simulink model "Controlled_Motor_Position"  (R2020b)
settings: Solver=VariableStepAuto  StartTime=0.0  StopTime=10.0  RelTol=1e-3
values from neighbouring files (symbols this model uses):
  b = 3.5077E-6    [data.sldd]
  J = 3.2284E-6    [data.sldd]
  K = 0.0274    [data.sldd]
  Kd = 0.04    [data.sldd]
  Ki = 47.4    [data.sldd]
  Kp = 3.4    [data.sldd]
  L = 2.75E-6    [data.sldd]
  R = 4.0    [data.sldd]
settings Model: DataDictionary=data.sldd  Creator=vikas  LastModifiedBy=family

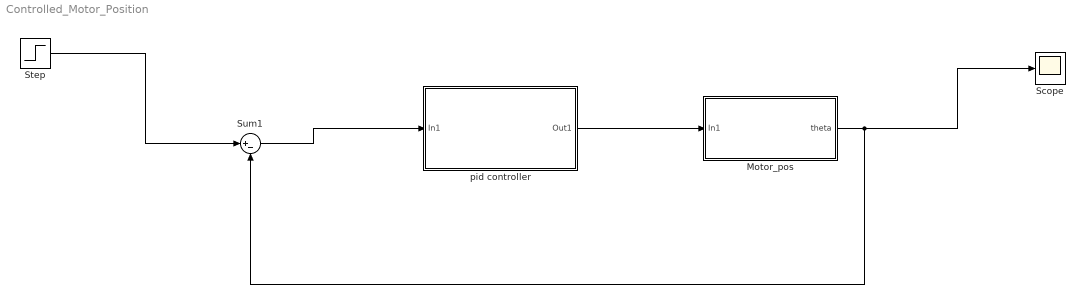
== system Controlled_Motor_Position ==
  Motor_pos : Subsystem
  Scope : Scope
  Step : Step  SampleTime=0
  Sum1 : Sum  Inputs=|+-
  pid controller : Subsystem
  wires:
  Step/1 -> Sum1/1
  Sum1/1 -> pid controller/1(In1)
  Motor_pos/1(theta) -> Scope/1, Sum1/2
  pid controller/1(Out1) -> Motor_pos/1(In1)

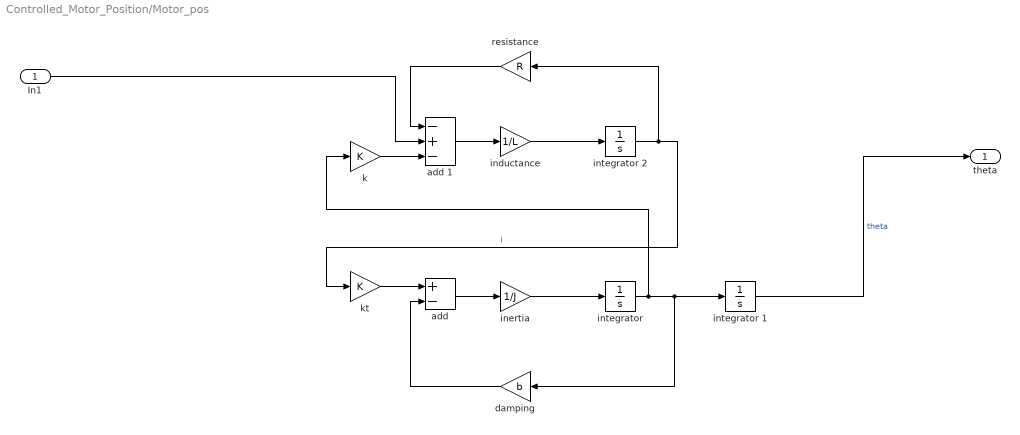
== system Controlled_Motor_Position/Motor_pos ==
  In1 : Inport
  add : Sum  Inputs=+-
  add 1 : Sum  Inputs=-+-
  damping : Gain  Gain=b
  inductance : Gain  Gain=1/L
  inertia : Gain  Gain=1/J
  integrator : Integrator
  integrator 1 : Integrator
  integrator 2 : Integrator
  k : Gain  Gain=K
  kt : Gain  Gain=K
  resistance : Gain  Gain=R
  theta : Outport
  wires:
  damping/1 -> add/2
  integrator 2/1 -> kt/1, resistance/1  "i"
  k/1 -> add 1/3
  integrator/1 -> k/1, damping/1, integrator 1/1
  kt/1 -> add/1
  inertia/1 -> integrator/1
  add 1/1 -> inductance/1
  add/1 -> inertia/1
  inductance/1 -> integrator 2/1
  integrator 1/1 -> theta/1  "theta"
  resistance/1 -> add 1/1
  In1/1 -> add 1/2

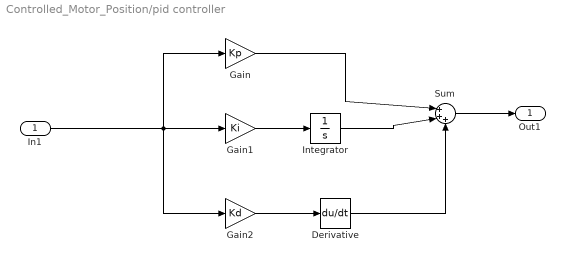
== system Controlled_Motor_Position/pid controller ==
  In1 : Inport
  Derivative : Derivative
  Gain : Gain  Gain=Kp
  Gain1 : Gain  Gain=Ki
  Gain2 : Gain  Gain=Kd
  Integrator : Integrator
  Sum : Sum  Inputs=|+++
  Out1 : Outport
  wires:
  Gain1/1 -> Integrator/1
  In1/1 -> Gain2/1, Gain/1, Gain1/1
  Derivative/1 -> Sum/3
  Integrator/1 -> Sum/2
  Gain/1 -> Sum/1
  Gain2/1 -> Derivative/1
  Sum/1 -> Out1/1
